simulink model "siasun_config_casadi_VS_lsj_sim_16a"  (R2020a)
settings: Solver=FixedStepAuto  StartTime=0.0  StopTime=20  FixedStep=0.001  RelTol=1e-3  EnableMultiTasking=on
values from neighbouring files (symbols this model uses):
  a1 = 0.040    (= 0.04)    [set_mode_parameter_siasun.m]
  a2 = 0.275    [set_mode_parameter_siasun.m]
  a3 = 0.025    [set_mode_parameter_siasun.m]
  d1 = 0.342    [set_mode_parameter_siasun.m]
  d4 = 0.280    (= 0.28)    [set_mode_parameter_siasun.m]
  fc1 = 0    [set_mode_parameter_siasun.m]
  fc2 = 0    [set_mode_parameter_siasun.m]
  fc3 = 0    [set_mode_parameter_siasun.m]
  fc4 = 0    [set_mode_parameter_siasun.m]
  fc5 = 0    [set_mode_parameter_siasun.m]
  fc6 = 0    [set_mode_parameter_siasun.m]
  fv1 = 0    [set_mode_parameter_siasun.m]
  fv2 = 0    [set_mode_parameter_siasun.m]
  fv3 = 0    [set_mode_parameter_siasun.m]
  fv4 = 0    [set_mode_parameter_siasun.m]
  fv5 = 0    [set_mode_parameter_siasun.m]
  fv6 = 0    [set_mode_parameter_siasun.m]
  Ia1 = 0    [set_mode_parameter_siasun.m]
  Ia2 = 0    [set_mode_parameter_siasun.m]
  Ia3 = 0    [set_mode_parameter_siasun.m]
  Ia4 = 0    [set_mode_parameter_siasun.m]
  Ia5 = 0    [set_mode_parameter_siasun.m]
  Ia6 = 0    [set_mode_parameter_siasun.m]
  Ic111 = 0    [set_mode_parameter_siasun.m]
  Ic112 = 0    [set_mode_parameter_siasun.m]
  Ic113 = 0    [set_mode_parameter_siasun.m]
  Ic122 = 0    [set_mode_parameter_siasun.m]
  Ic123 = 0    [set_mode_parameter_siasun.m]
  Ic133 = 1.3676    [set_mode_parameter_siasun.m]
  Ic211 = 8.8194    [set_mode_parameter_siasun.m]
  Ic212 = 0    [set_mode_parameter_siasun.m]
  Ic213 = 0    [set_mode_parameter_siasun.m]
  Ic222 = 6.0549    [set_mode_parameter_siasun.m]
  Ic223 = 0    [set_mode_parameter_siasun.m]
  Ic233 = 0.9569    [set_mode_parameter_siasun.m]
  Ic311 = 0.0332    [set_mode_parameter_siasun.m]
  Ic312 = 0    [set_mode_parameter_siasun.m]
  Ic313 = 0    [set_mode_parameter_siasun.m]
  Ic322 = 1.8442    [set_mode_parameter_siasun.m]
  Ic323 = 0    [set_mode_parameter_siasun.m]
  Ic333 = 1.0560    (= 1.056)    [set_mode_parameter_siasun.m]
  Ic411 = 0.1448    [set_mode_parameter_siasun.m]
  Ic412 = 0    [set_mode_parameter_siasun.m]
  Ic413 = 0    [set_mode_parameter_siasun.m]
  Ic422 = 0.0015    [set_mode_parameter_siasun.m]
  Ic423 = 0    [set_mode_parameter_siasun.m]
  Ic433 = 0.0822    [set_mode_parameter_siasun.m]
  Ic511 = 0    [set_mode_parameter_siasun.m]
  Ic512 = 0    [set_mode_parameter_siasun.m]
  Ic513 = 0    [set_mode_parameter_siasun.m]
  Ic522 = 0.0121    [set_mode_parameter_siasun.m]
  Ic523 = 0    [set_mode_parameter_siasun.m]
  Ic533 = 0.0299    [set_mode_parameter_siasun.m]
  Ic611 = 0.0134    [set_mode_parameter_siasun.m]
  Ic612 = 0    [set_mode_parameter_siasun.m]
  Ic613 = 0    [set_mode_parameter_siasun.m]
  Ic622 = 0    [set_mode_parameter_siasun.m]
  Ic623 = 0    [set_mode_parameter_siasun.m]
  Ic633 = 0.0051    [set_mode_parameter_siasun.m]
  m1 = 0.167    [set_mode_parameter_siasun.m]
  m2 = 1    [set_mode_parameter_siasun.m]
  m3 = 0.5    [set_mode_parameter_siasun.m]
  m4 = 0.333    [set_mode_parameter_siasun.m]
  m5 = 0.25    [set_mode_parameter_siasun.m]
  m6 = 0.2    [set_mode_parameter_siasun.m]
  mc11 = 0    [set_mode_parameter_siasun.m]
  mc12 = 0    [set_mode_parameter_siasun.m]
  mc13 = 0.2    [set_mode_parameter_siasun.m]
  mc21 = 0.1291    [set_mode_parameter_siasun.m]
  mc22 = 0    [set_mode_parameter_siasun.m]
  mc23 = 3.3117    [set_mode_parameter_siasun.m]
  mc31 = 1.6484    [set_mode_parameter_siasun.m]
  mc32 = 0    [set_mode_parameter_siasun.m]
  mc33 = 0.8748    [set_mode_parameter_siasun.m]
  mc41 = 0.3200    (= 0.32)    [set_mode_parameter_siasun.m]
  mc42 = 0.2324    [set_mode_parameter_siasun.m]
  mc43 = 0.7083    [set_mode_parameter_siasun.m]
  mc51 = 0.4574    [set_mode_parameter_siasun.m]
  mc52 = 0    [set_mode_parameter_siasun.m]
  mc53 = 0.6427    [set_mode_parameter_siasun.m]
  mc61 = 0.3200    (= 0.32)    [set_mode_parameter_siasun.m]
  mc62 = -0.0513    [set_mode_parameter_siasun.m]
  mc63 = 0.6417    [set_mode_parameter_siasun.m]
undefined symbols (not defined in the file or in its folder): X, Y, Z
libraries: sm_lib x224, nesl_utility x124, simulink x8
(part 7 of 11)

== matlab function siasun_config_casadi_VS_lsj_sim_16a/Cartesian_trajectory1 ==
  data: time input; q output; initq output
function [q,initq]  = Cartesian(time)
    
    % 每次运行之前改变一下间距，再重新运行
    S = load('path.mat');
    %%  traj - 6xn
    traj = S.path;
